simulink model "EEG_Record"  (R2014a)
settings: Solver=FixedStepDiscrete  StartTime=0.0  StopTime=inf  FixedStep=1/256  RelTol=1e-3  EnableMultiTasking=on
InitFcn:
  | set_param('EEG_Record/Subsystem1/Gain1','Gain','0');
  | set_param('EEG_Record/Stop_Simulation','value','0');
  | 
  | ts=1/256;
StartFcn:
  | ParadigmStart;
undefined symbols (not defined in the file or in its folder): currentCFG_EEG_Record_UA, UA
libraries: Tools x2, gUSBamplib x1
settings Model: Creator=BIOLABB  LastModifiedBy=PC
settings OptimizationCC: BlockReduction=off  BooleanDataType=off  SimCompilerOptimization=off
settings DebuggingCC: SaveWithParameterizedLinksMsg=none  UnderspecifiedInitializationDetection=Classic  SignalResolutionControl=TryResolveAllWithWarning  SolverPrmCheckMsg=none  FcnCallInpInsideContextMsg=error  FrameProcessingCompatibilityMsg=error  SFExecutionAtInitializationDiag=none
settings HardwareCC: ProdBitPerSizeT=32  ProdBitPerPtrDiffT=32  TargetUnknown=on
settings RTWCC: RTWCompilerOptimization=off
settings ConfigComp: CovMetricSettings=dw  CovHtmlReporting=on  CovSaveCumulativeToWorkspaceVar=on  CovSaveSingleToWorkspaceVar=on  CovExternalEMLEnable=off  CovSFcnEnable=off

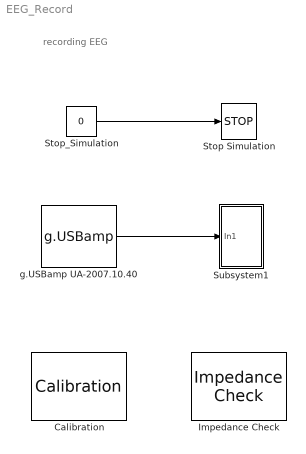
== system EEG_Record ==
  note: recording EEG
  Calibration : Tools/Calibration  SystemSampleTime=-1
  Impedance Check : Tools/Impedance Check  SystemSampleTime=-1
  Stop Simulation : Stop
  Stop_Simulation : Constant  Value=0  SampleTime=ts
  Subsystem1 : Subsystem
  g.USBamp UA-2007.10.40 : gUSBamplib/g.USBamp  Priority=2  cfg=currentCFG_EEG_Record_UA-2007.10.40.cfg  snr=UA-2007.10.40
  wires:
  g.USBamp UA-2007.10.40/1 -> Subsystem1/1(In1)
  Stop_Simulation/1 -> Stop Simulation/1

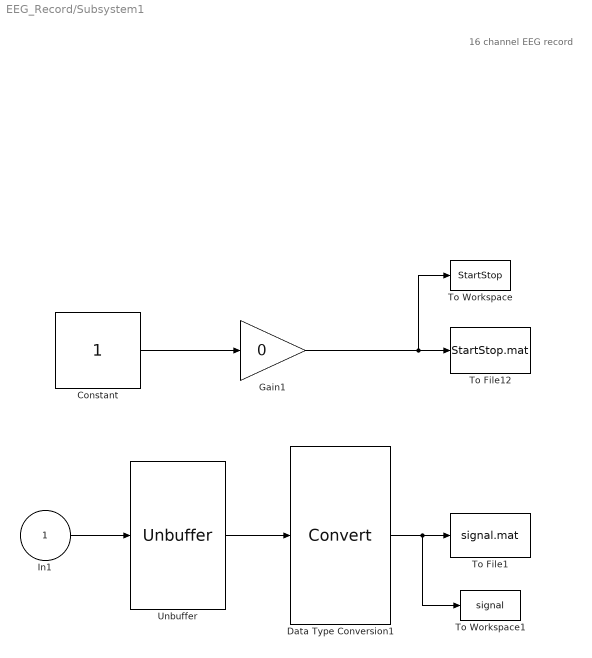
== system EEG_Record/Subsystem1 ==
  note: 16 channel EEG record
  In1 : Inport
  Constant : Constant
  Data Type Conversion1 : DataTypeConversion  SampleTime=ts  SaturateOnIntegerOverflow=on  RndMeth=Zero
  Gain1 : Gain  Gain=0
  To File1 : ToFile  Filename=signal.mat  MatrixName=signal  SampleTime=ts
  To File12 : ToFile  Filename=StartStop.mat  MatrixName=StartStop  SampleTime=ts
  To Workspace : ToWorkspace  VariableName=StartStop  SampleTime=ts
  To Workspace1 : ToWorkspace  VariableName=signal  SampleTime=ts
  Unbuffer : Unbuffer
  wires:
  Data Type Conversion1/1 -> To Workspace1/1, To File1/1
  Gain1/1 -> To Workspace/1, To File12/1
  Constant/1 -> Gain1/1
  Unbuffer/1 -> Data Type Conversion1/1
  In1/1 -> Unbuffer/1
